simulink model "controller_3_3"  (R2023b)
settings: Solver=VariableStepAuto  StartTime=0.0  StopTime=10.0  RelTol=1e-3
settings Model: Creator=sarth  LastModifiedBy=sarth

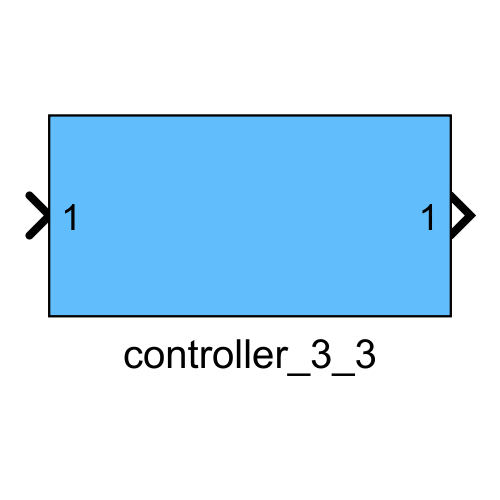
[thumbnail: Simulink's stored preview of the top-level diagram]
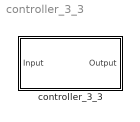
== system controller_3_3 ==
  controller_3_3 : Subsystem

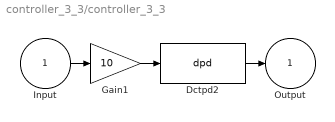
== system controller_3_3/controller_3_3 ==
  Input : Inport
  Dctpd2 : S-Function  FunctionName=dpd  Parameters=kp, kv, 0.001  SFunctionDeploymentMode=off  EnableBusSupport=off  mask(dctools){kp=2.5, kv=0.01}
      mask help: This block implements a discrete time pd filter.
      mask Display: disp('DCT pd')
  Gain1 : Gain  Gain=10
  Output : Outport
  wires:
  Input/1 -> Gain1/1
  Gain1/1 -> Dctpd2/1
  Dctpd2/1 -> Output/1
